simulink model "Speed_Control_SVPWM"  (R2023b)
settings: Solver=ode3  StartTime=0.0  StopTime=10  FixedStep=1e-5  RelTol=1e-3
undefined symbols (not defined in the file): DiscIntNeverNeededParam
libraries: spsIGBTDiodeLib x6, spsCurrentMeasurementLib x3, spsAsynchronousMachineSIUnitsLib x1, spsDCVoltageSourceLib x1, slpidlib x1, simulink x1, sps_lib x1
settings Model: Creator=G Nithish Chandra  LastModifiedBy=G Nithish Chandra

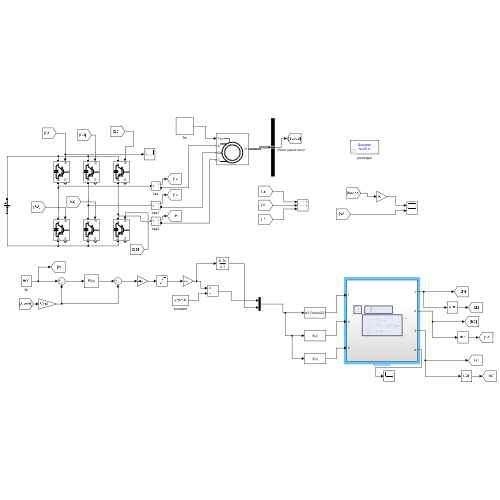
[thumbnail: Simulink's stored preview of the top-level diagram]
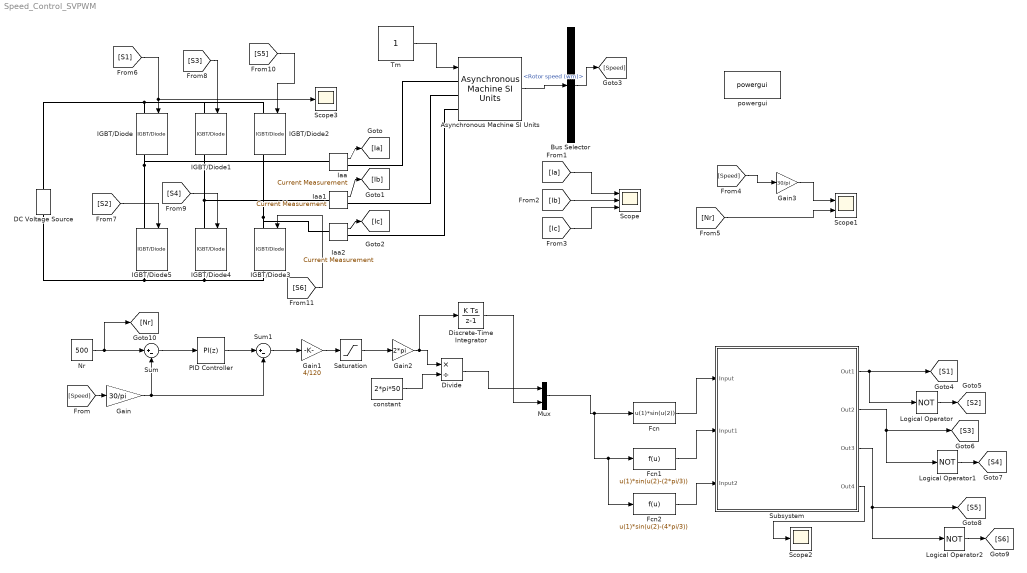
== system Speed_Control_SVPWM ==
  Asynchronous Machine SI Units : spsAsynchronousMachineSIUnitsLib/Asynchronous Machine SI Units  RotorType=Squirrel-cage  PresetModel="01:  5 HP   460 V 60Hz 1750 RPM"  MechanicalLoad=Torque Tm  ShowDetailedParameters=on  ReferenceFrame=Rotor  Units=SI  MeasurementBus=off  NominalParameters=[3730 460 60]  VoltageRatio=1  Stator=[1.115 0.005974]  Rotor=[1.083 0.005974]  Cage1=[0.4155 0.002066]  Cage2=[0.4168 0.0003495]  Lm=0.2037  Mechanical=[0.02 0.005752 2]  PolePairs=2  InitialConditions=[0 0 0 0 0 0 0 0]  SimulateSaturation=off  Saturation=[14.03593122, 27.81365428, 53.79336849, 72.68890987, 97.98006896, 148.6815601, 215.7428561, 302.9841135, 428.7778367 ; 230, 322, 414, 460, 506, 552, 598, 644, 690]  LoadFlowParameters=1492000  TsPowergui=0  TsBlock=-1  IterativeModel=Trapezoidal non iterative  IterativeDiscreteModel=Trapezoidal non iterative  Pmec=1.492e+006
  Bus Selector : BusSelector  OutputSignals=Mechanical.Rotor speed (wm)
  DC Voltage Source : spsDCVoltageSourceLib/DC Voltage Source  Amplitude=572  Measurements=Voltage
  Discrete-Time Integrator : DiscreteIntegrator  SampleTime=-1  ICPrevOutput=DiscIntNeverNeededParam  ICPrevScaledInput=DiscIntNeverNeededParam
  Divide : Product  Inputs=*/
  Fcn : Fcn  Expr=u(1)*sin(u(2))
  Fcn1 : Fcn  Expr=u(1)*sin(u(2)-(2*pi/3))
  Fcn2 : Fcn  Expr=u(1)*sin(u(2)-(4*pi/3))
  Gain : Gain  Gain=30/pi
  Gain1 : Gain  Gain=4/120
  Gain2 : Gain  Gain=2*pi
  Gain3 : Gain  Gain=30/pi
  IGBT/Diode{,1..5} (6 alike) : spsIGBTDiodeLib/IGBT//Diode  Ron=1e-3  Rs=1e5  Cs=inf  Measurements=on
  Iaa : spsCurrentMeasurementLib/Current Measurement  PhasorSimulation=off  OutputType=Complex  PSBequivalent=0
  Iaa1 : spsCurrentMeasurementLib/Current Measurement  PhasorSimulation=off  OutputType=Complex  PSBequivalent=0
  Iaa2 : spsCurrentMeasurementLib/Current Measurement  PhasorSimulation=off  OutputType=Complex  PSBequivalent=0
  Logical Operator : Logic  Operator=NOT  AllPortsSameDT=off  OutDataTypeStr=boolean
  Logical Operator1 : Logic  Operator=NOT  AllPortsSameDT=off  OutDataTypeStr=boolean
  Logical Operator2 : Logic  Operator=NOT  AllPortsSameDT=off  OutDataTypeStr=boolean
  Mux : Mux  Inputs=2
  Nr : Constant  Value=500
  PID Controller : slpidlib/PID Controller  Controller=PI  Form=Parallel  TimeDomain=Discrete-time  UseExternalTs=off  SampleTime=-1  IntegratorMethod=Forward Euler  FilterMethod=Forward Euler  ControllerParametersSource=internal  P=1  I=10  UseKiTs=off  D=0  N=100  UseFilter=on  TunerSelectOption=Transfer Function Based (PID Tuner App)  InitialConditionSource=internal  InitialConditionForIntegrator=0  InitialConditionForFilter=0  DifferentiatorICPrevScaledInput=0  ExternalReset=none  TrackingMode=off  Kt=1  LimitOutput=off  SatLimitsSource=internal  UpperSaturationLimit=inf  LowerSaturationLimit=-inf  LinearizeAsGain=on  AntiWindupMode=none  Kb=1  LimitIntegrator=off  UpperIntegratorSaturationLimit=inf  LowerIntegratorSaturationLimit=-inf  POutMin=[]  POutMax=[]  IOutMin=[]  IOutMax=[]  DOutMin=[]  DOutMax=[]  NOutMin=[]  NOutMax=[]  SumOutMin=[]  SumOutMax=[]  SaturationOutMin=[]  SaturationOutMax=[]  PParamMin=[]  PParamMax=[]  IParamMin=[]  IParamMax=[]  DParamMin=[]  DParamMax=[]  NParamMin=[]  NParamMax=[]  KbParamMin=[]  KbParamMax=[]  KtParamMin=[]  KtParamMax=[]  KbOutMin=[]  KbOutMax=[]  KtOutMin=[]  KtOutMax=[]  IntegratorOutMin=[]  IntegratorOutMax=[]  FilterOutMin=[]  FilterOutMax=[]  SumI1OutMin=[]  SumI1OutMax=[]  SumI2OutMin=[]  SumI2OutMax=[]  SumI3OutMin=[]  SumI3OutMax=[]  SumI4OutMin=[]  SumI4OutMax=[]  SumDOutMin=[]  SumDOutMax=[]  DifferentiatorOutMin=[]  DifferentiatorOutMax=[]  FilterDiffOutCoefMin=[]  FilterDiffOutCoefMax=[]  ReciprocalOutMin=[]  ReciprocalOutMax=[]  SumDenOutMin=[]  SumDenOutMax=[]  SumNumOutMin=[]  SumNumOutMax=[]  DivideOutMin=[]  DivideOutMax=[]  UdiffTsProdOutMin=[]  UdiffTsProdOutMax=[]  NTsProdOutMin=[]  NTsProdOutMax=[]  UintegralTsProdOutMin=[]  UintegralTsProdOutMax=[]  UngainTsProdOutMin=[]  UngainTsProdOutMax=[]  ClampingZeroOutDataTypeStr=Inherit: Inherit via back propagation  ClampingZeroOutMin=[]  ClampingZeroOutMax=[]  FilterDenConstantOutDataTypeStr=Inherit: Inherit via back propagation  FilterDenConstantOutMin=[]  FilterDenConstantOutMax=[]  PCopyOutDataTypeStr=Inherit: Inherit via back propagation  PCopyOutMin=[]  PCopyOutMax=[]  NCopyOutDataTypeStr=Inherit: Inherit via back propagation  NCopyOutMin=[]  NCopyOutMax=[]  IntegratorContinuousStateAttributes=''  IntegratorStateMustResolveToSignalObject=off  IntegratorRTWStateStorageClass=Auto  FilterContinuousStateAttributes=''  FilterStateMustResolveToSignalObject=off  FilterRTWStateStorageClass=Auto  ParallelPVariant=InternalParameters  IdealPVariant=Disabled  IVariant=InternalParameters  DVariant=Disabled  IntegratorVariant=Discrete  SatVariant=Disabled  AWVariant=Passthrough  PCopyVariant=Disabled  TRVariant=Disabled  FdbkBlocksVariant=Forward  IdealPFdbkVariant=Disabled  SatFdbkVariant=Disabled  DerivativeFilterVariant=Disabled  NVariant=Disabled  NCopyVariant=Disabled_SignalSpec  FilterICVariant=Disabled  IntegratorICVariant=InternalICs  ExternalResetVariant=Disabled  TRSumVariant=Passthrough  SumFdbkVariant=Disabled  SumVariant=Sum_PI  TsampFilterVariant=InternalTs  TsampNgainVariant=Passthrough  TsampIntegralVariant=Disabled_SignalSpec  ExternalSaturationOutDataTypeStr=Inherit: Same as second input
  Saturation : Saturate  UpperLimit=50  LowerLimit=0
  Scope : Scope  NumInputPorts=3
  Scope1 : Scope  NumInputPorts=2
  Scope2 : Scope
  Scope3 : Scope
  Subsystem : Subsystem
  Sum : Sum  Inputs=|+-
  Sum1 : Sum  Inputs=|+-
  Tm : Constant
  constant : Constant  Value=2*pi*50
  powergui : sps_lib/powergui  Priority=1  SimulationMode=Discrete  SampleTime=1e-5  frequency=60  Iterations=50  frequencyindice=60  Pbase=100e6  ErrMax=1e-4  UnitsV=kV  UnitsW=MW  buscounter=0  FunctionMessages=off  echomessages=off  EnableUseOfTLC=off  CurrentSourceSwitches=off  DisableSnubberDevices=off  DisableRonSwitches=off  DisableVfSwitches=off  DisplayEquations=off  AutomaticDiscreteSolvers=off  SolverType=Tustin  Interpol=off  ExternalGateDelay=off  methode=off  Ts=100  x0status=blocks  SPID=on  SwTol=0  HookPort=off  NonlinearTolerance=1e-4  nMaxIteration=100  ContinueOnMaxIteration=off  RestoreLinks=warning  ResistiveCurrentMeasurement=off  Frange=[0:2:500]  Ylog=off  Xlog=on  ShowGrid=off  save=off  variable=ZData  structure=0  ZoomFFT=off  StartTime=0.0  cycles=1  DisplayStyle=1  fundamental=60  FreqAxis=off  MaxFrequency=1000  frequencyindicesteady=1  RmsSteady=1  display=off
  wires:
  Iaa/1 -> [Ia]
  Iaa1/1 -> [Ib]
  Iaa2/1 -> [Ic]
  Tm/1 -> Asynchronous Machine SI Units/1
  Asynchronous Machine SI Units/1 -> Bus Selector/1
  Bus Selector/1 -> [Speed]  "<Rotor speed (wm)>"
  [Speed] -> Gain/1
  Gain/1 -> Sum1/2, Sum/2
  Nr/1 -> [Nr], Sum/1
  Sum/1 -> PID Controller/1
  PID Controller/1 -> Sum1/1
  Sum1/1 -> Gain1/1
  Gain1/1 -> Saturation/1
  Saturation/1 -> Gain2/1
  Gain2/1 -> Discrete-Time Integrator/1, Divide/1
  constant/1 -> Divide/2
  Fcn/1 -> Subsystem/1(Input)
  Fcn1/1 -> Subsystem/2(Input1)
  Fcn2/1 -> Subsystem/3(Input2)
  Subsystem/1(Out1) -> Logical Operator/1, [S1]
  Logical Operator/1 -> [S2]
  Logical Operator1/1 -> [S4]
  Subsystem/2(Out2) -> Logical Operator1/1, [S3]
  Subsystem/3(Out3) -> [S5], Logical Operator2/1
  Logical Operator2/1 -> [S6]
  [Ia] -> Scope/1
  [Ib] -> Scope/2
  [Ic] -> Scope/3
  [Speed] -> Gain3/1
  Gain3/1 -> Scope1/1
  [Nr] -> Scope1/2
  Discrete-Time Integrator/1 -> Mux/2
  Divide/1 -> Mux/1
  Mux/1 -> Fcn2/1, Fcn1/1, Fcn/1
  [S1] -> Scope3/1, IGBT/Diode/1
  [S3] -> IGBT/Diode1/1
  [S5] -> IGBT/Diode2/1
  [S2] -> IGBT/Diode5/1
  [S4] -> IGBT/Diode4/1
  [S6] -> IGBT/Diode3/1
  Subsystem/4(Out4) -> Scope2/1
  connections:
  IGBT/Diode/LConn1 -- IGBT/Diode1/LConn1 -- IGBT/Diode2/LConn1 -- DC Voltage Source/RConn1
  Iaa/RConn1 -- Asynchronous Machine SI Units/LConn1
  Iaa1/RConn1 -- Asynchronous Machine SI Units/LConn2
  Iaa2/RConn1 -- Asynchronous Machine SI Units/LConn3
  IGBT/Diode5/LConn1 -- Iaa/LConn1 -- IGBT/Diode/RConn1
  IGBT/Diode1/RConn1 -- Iaa1/LConn1 -- IGBT/Diode4/LConn1
  IGBT/Diode2/RConn1 -- Iaa2/LConn1 -- IGBT/Diode3/LConn1
  IGBT/Diode5/RConn1 -- IGBT/Diode3/RConn1 -- IGBT/Diode4/RConn1 -- DC Voltage Source/LConn1

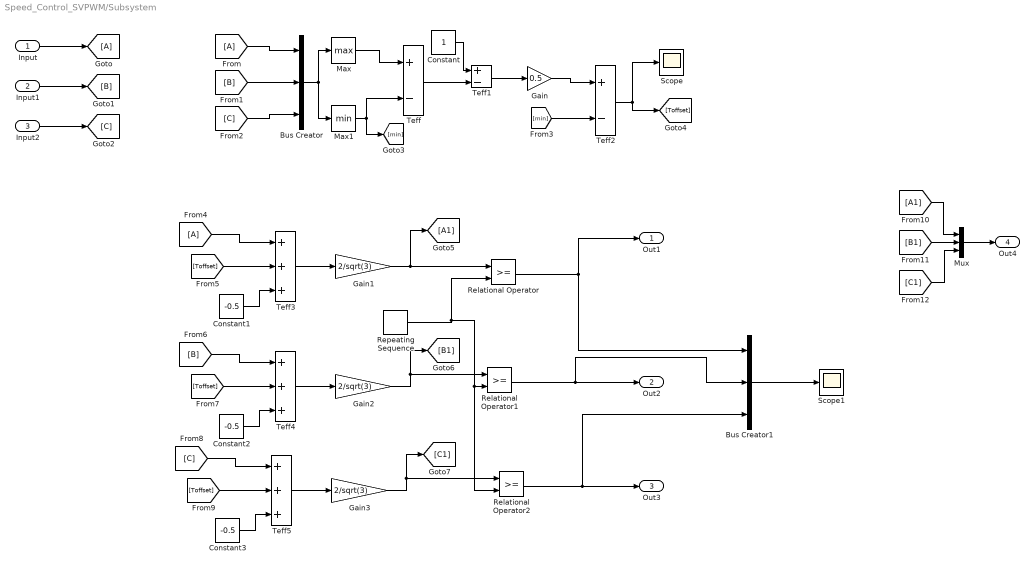
== system Speed_Control_SVPWM/Subsystem ==
  Input : Inport
  Input1 : Inport  Port=2
  Input2 : Inport  Port=3
  Bus Creator : BusCreator  Inputs=3
  Bus Creator1 : BusCreator  Inputs=3
  Constant : Constant
  Constant1 : Constant  Value=-0.5
  Constant2 : Constant  Value=-0.5
  Constant3 : Constant  Value=-0.5
  From : From
  From4 : From
  Gain : Gain  Gain=0.5
  Gain1 : Gain  Gain=2/sqrt(3)
  Gain2 : Gain  Gain=2/sqrt(3)
  Gain3 : Gain  Gain=2/sqrt(3)
  Goto : Goto
  Max : MinMax  Function=max
  Max1 : MinMax
  Mux : Mux  Inputs=3
  Relational Operator : RelationalOperator  OutDataTypeStr=boolean  RndMeth=Simplest  InputSameDT=off
  Relational Operator1 : RelationalOperator  OutDataTypeStr=boolean  RndMeth=Simplest  InputSameDT=off
  Relational Operator2 : RelationalOperator  OutDataTypeStr=boolean  RndMeth=Simplest  InputSameDT=off
  Repeating Sequence : simulink/Sources/Repeating Sequence  rep_seq_t=[0 1 2]*(1/4100)  rep_seq_y=[-1 1 -1]
  Scope : Scope
  Scope1 : Scope
  Teff : Sum  Inputs=+-
  Teff1 : Sum  Inputs=+-
  Teff2 : Sum  Inputs=+-
  Teff3 : Sum  Inputs=+++
  Teff4 : Sum  Inputs=+++
  Teff5 : Sum  Inputs=+++
  Out1 : Outport
  Out2 : Outport  Port=2
  Out3 : Outport  Port=3
  Out4 : Outport  Port=4
  wires:
  Input/1 -> Goto/1
  Input1/1 -> [B]
  Input2/1 -> [C]
  From/1 -> Bus Creator/1
  [B] -> Bus Creator/2
  [C] -> Bus Creator/3
  Bus Creator/1 -> Max1/1, Max/1
  Max/1 -> Teff/1
  Max1/1 -> [min], Teff/2
  Constant/1 -> Teff1/1
  Teff/1 -> Teff1/2
  Teff1/1 -> Gain/1
  Gain/1 -> Teff2/1
  [min] -> Teff2/2
  Teff2/1 -> [Toffset], Scope/1
  From4/1 -> Teff3/1
  [Toffset] -> Teff3/2
  Constant1/1 -> Teff3/3
  Teff3/1 -> Gain1/1
  Gain1/1 -> Relational Operator/1, [A1]
  Repeating Sequence/1 -> Relational Operator2/2, Relational Operator1/2, Relational Operator/2
  Relational Operator/1 -> Bus Creator1/1, Out1/1
  Gain2/1 -> Relational Operator1/1, [B1]
  Teff4/1 -> Gain2/1
  Constant2/1 -> Teff4/3
  [Toffset] -> Teff4/2
  [B] -> Teff4/1
  [C] -> Teff5/1
  [Toffset] -> Teff5/2
  Constant3/1 -> Teff5/3
  Teff5/1 -> Gain3/1
  Gain3/1 -> Relational Operator2/1, [C1]
  Relational Operator1/1 -> Bus Creator1/2, Out2/1
  Relational Operator2/1 -> Out3/1, Bus Creator1/3
  Bus Creator1/1 -> Scope1/1
  [A1] -> Mux/1
  [B1] -> Mux/2
  [C1] -> Mux/3
  Mux/1 -> Out4/1
